simulink model "rl_pwm"  (R2020b)
settings: Solver=ode45  StartTime=0.0  StopTime=0.2  RelTol=1e-3  EnableMultiTasking=on
values from neighbouring files (symbols this model uses):
  E = 10    [task1.m]
  L = 0.05    [task1.m]
  R = 2    [task1.m]
  Ts = 0.002    [task1.m]
  Udc = 600    [task1.m]
settings Model: Creator=ielolof  LastModifiedBy=axelfroborg
settings DataIOCC: SaveFormat=Array  SignalLoggingSaveFormat=ModelDataLogs  ReturnWorkspaceOutputs=off  TimeSaveName=tpwm
settings OptimizationCC: ExpressionDepthLimit=2147483647  InitFltsAndDblsToZero=on  LifeSpan=inf
settings DebuggingCC: UnderspecifiedInitializationDetection=Classic  MergeDetectMultiDrivingBlocksExec=none  SolverPrmCheckMsg=warning  FcnCallInpInsideContextMsg=warning  StateNameClashWarn=warning  SFUnexpectedBacktrackingDiag=warning  SFNoUnconditionalDefaultTransitionDiag=warning  SFExecutionAtInitializationDiag=none  ArithmeticOperatorsInVariantConditions=warning
settings HardwareCC: ProdBitPerPointer=32  ProdBitPerSizeT=32  ProdBitPerPtrDiffT=32  ProdLargestAtomicFloat=None  ProdIntDivRoundTo=Undefined  ProdEndianess=Unspecified  ProdWordSize=32  ProdHWDeviceType=32-bit Generic
settings ModelReferenceCC: PropagateSignalLabelsOutOfModel=off
settings SFSimCC: SimUseLocalCustomCode=off  CustomCodeUndefinedFunction=UseInterfaceOnly
settings RTWCC: RTWUseLocalCustomCode=off
settings CodeAppCC: StateflowObjectComments=on
settings GRTTargetCC: TargetLangStandard=C89/C90 (ANSI)  CombineOutputUpdateFcns=off  GRTInterface=on
settings ConfigComp: CovMetricSettings=dw  CovSaveCumulativeToWorkspaceVar=on  CovSaveSingleToWorkspaceVar=on  CovExternalEMLEnable=off

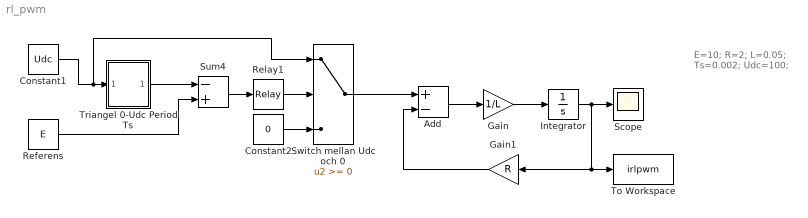
== system rl_pwm ==
  note: E=10;
      | R=2;
      | L=0.05;
      |
      | Ts=0.002;
      | Udc=100;
  Add : Sum  Inputs=+-
  Constant1 : Constant  Value=Udc
  Constant2 : Constant  Value=0
  Gain : Gain  Gain=1/L
  Gain1 : Gain  Gain=R
  Integrator : Integrator
  Referens : Constant  Value=E
  Relay1 : Relay  OffOutputValue=-1
  Scope : Scope
  Sum4 : Sum  Inputs=-+  InputSameDT=on  SaturateOnIntegerOverflow=on  OutDataTypeStr=Inherit: Same as first input
  Switch mellan Udc och 0 : Switch  SaturateOnIntegerOverflow=on  InputSameDT=on
  To Workspace : ToWorkspace  VariableName=irlpwm  SampleTime=-1
  Triangel 0-Udc Period Ts : Subsystem
  wires:
  Constant1/1 -> Switch mellan Udc och 0/1, Triangel 0-Udc Period Ts/1(Udc)
  Triangel 0-Udc Period Ts/1(um) -> Sum4/1
  Sum4/1 -> Relay1/1
  Gain1/1 -> Add/2
  Add/1 -> Gain/1
  Gain/1 -> Integrator/1
  Integrator/1 -> Gain1/1, To Workspace/1, Scope/1
  Switch mellan Udc och 0/1 -> Add/1
  Referens/1 -> Sum4/2
  Relay1/1 -> Switch mellan Udc och 0/2
  Constant2/1 -> Switch mellan Udc och 0/3

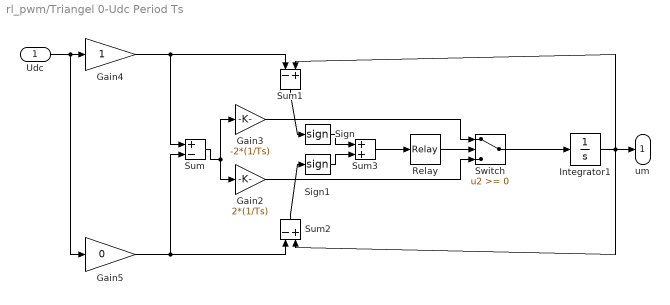
== system rl_pwm/Triangel 0-Udc Period Ts ==
  Udc : Inport
  Gain2 : Gain  Gain=2*(1/Ts)  SaturateOnIntegerOverflow=on  OutDataTypeStr=Inherit: Same as input  ParamDataTypeStr=Inherit: Same as input
  Gain3 : Gain  Gain=-2*(1/Ts)  SaturateOnIntegerOverflow=on  OutDataTypeStr=Inherit: Same as input  ParamDataTypeStr=Inherit: Same as input
  Gain4 : Gain  SaturateOnIntegerOverflow=on  OutDataTypeStr=Inherit: Same as input  ParamDataTypeStr=Inherit: Same as input
  Gain5 : Gain  Gain=0  SaturateOnIntegerOverflow=on  OutDataTypeStr=Inherit: Same as input  ParamDataTypeStr=Inherit: Same as input
  Integrator1 : Integrator
  Relay : Relay  OnSwitchValue=1  OffSwitchValue=-1  OffOutputValue=-1
  Sign : Signum
  Sign1 : Signum
  Sum : Sum  Inputs=+-  InputSameDT=on  SaturateOnIntegerOverflow=on  OutDataTypeStr=Inherit: Same as first input
  Sum1 : Sum  Inputs=-+  InputSameDT=on  SaturateOnIntegerOverflow=on  OutDataTypeStr=Inherit: Same as first input
  Sum2 : Sum  Inputs=-+  InputSameDT=on  SaturateOnIntegerOverflow=on  OutDataTypeStr=Inherit: Same as first input
  Sum3 : Sum  InputSameDT=on  SaturateOnIntegerOverflow=on  OutDataTypeStr=Inherit: Same as first input
  Switch : Switch  SaturateOnIntegerOverflow=on  InputSameDT=on
  um : Outport  VectorParamsAs1DForOutWhenUnconnected=off
  wires:
  Switch/1 -> Integrator1/1
  Gain3/1 -> Switch/1
  Gain2/1 -> Switch/3
  Integrator1/1 -> Sum1/2, Sum2/2, um/1
  Sum1/1 -> Sign/1
  Sum2/1 -> Sign1/1
  Sign/1 -> Sum3/1
  Sign1/1 -> Sum3/2
  Sum3/1 -> Relay/1
  Relay/1 -> Switch/2
  Sum/1 -> Gain3/1, Gain2/1
  Udc/1 -> Gain5/1, Gain4/1
  Gain5/1 -> Sum/2, Sum2/1
  Gain4/1 -> Sum/1, Sum1/1
